simulink model "recordEEGMultiVer"  (R2019a)
settings: Solver=VariableStepAuto  StartTime=0.0  StopTime=1000  RelTol=1e-3
undefined symbols (not defined in the file or in its folder): daq
libraries: dsparch4 x3, commrandsrc3 x3, daqlib x1, dspnetwork x1
settings Model: Creator=Kusunoki  LastModifiedBy=Owner

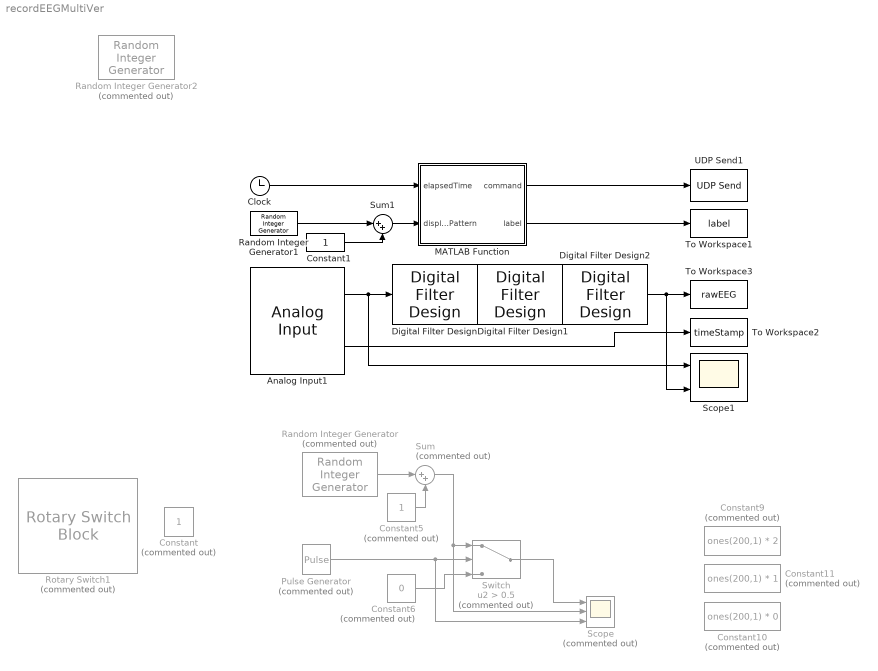
== system recordEEGMultiVer ==
  Analog Input1 : daqlib/Analog Input  DeviceMenu=ni Dev1 (USB-6000)  Device=ni Dev1 (USB-6000)  ObjConstructor=daq.createSession('ni')  NChannelsSelected=8  Channels=1$ai0$$Dev1$1$1$1$1$#1$ai1$$Dev1$1$1$1$1$#1$ai2$$Dev1$1$1$1$1$#1$ai3$$Dev1$1$1$1$1$#1$ai4$$Dev1$1$1$1$1$#1$ai5$$Dev1$1$1$1$1$#1$ai6$$Dev1$1$1$1$1$#1$ai7$$Dev1$1$1$1$1$#  NPorts=1 for all channels  SampleRate=1000  ActualRate=1000  ScansPerTrigger=200  OutputTimestamp=on  AcqMode=0  NumFrameBuffer=100  OutputTriggertime=off
      settings: SourceProductName=Data Acquisition Toolbox  SourceProductBaseCode=DA
  Clock : Clock
  Constant : Constant  Commented=on
  Constant1 : Constant
  Constant10 : Constant  Commented=on  Value=ones(200,1) * 0
  Constant11 : Constant  Commented=on  Value=ones(200,1) * 1
  Constant5 : Constant  Commented=on
  Constant6 : Constant  Commented=on  Value=0
  Constant9 : Constant  Commented=on  Value=ones(200,1) * 2
  Digital Filter Design : dsparch4/Digital Filter Design  mwdsp_browser_bugfix_var=off
  Digital Filter Design1 : dsparch4/Digital Filter Design  mwdsp_browser_bugfix_var=off
  Digital Filter Design2 : dsparch4/Digital Filter Design  mwdsp_browser_bugfix_var=off
  MATLAB Function : MATLAB Function  TreatAsAtomicUnit=on
  Pulse Generator : DiscretePulseGenerator  Commented=on  PulseType=Time based  Period=12  PulseWidth=10/12 * 100
  Random Integer Generator : commrandsrc3/Random Integer Generator  Commented=on  SetSize=2  SeedSource=Auto  Seed=0  SampleTime=12  SamplesPerFrame=1  OutputDataType=uint32  SimulateUsing=Interpreted execution
      settings: SourceProductName=Communications Toolbox
  Random Integer Generator1 : commrandsrc3/Random Integer Generator  SetSize=8  SeedSource=Auto  Seed=0  SampleTime=10  SamplesPerFrame=1  OutputDataType=uint32  SimulateUsing=Interpreted execution
      settings: SourceProductName=Communications Toolbox
  Random Integer Generator2 : commrandsrc3/Random Integer Generator  Commented=on  SetSize=3  SeedSource=Auto  Seed=0  SampleTime=3  SamplesPerFrame=1  OutputDataType=uint32  SimulateUsing=Interpreted execution
      settings: SourceProductName=Communications Toolbox
  Rotary Switch1 : RotarySwitchBlock  Commented=on
      settings: Values={{'0 : Relaxing', '1 : Gripping', '2 : Picking'}, [0 1 2]}
  Scope : Scope  Commented=on  NumInputPorts=3
  Scope1 : Scope  NumInputPorts=2
  Sum : Sum  Commented=on  Inputs=|++
  Sum1 : Sum  Inputs=|++
  Switch : Switch  Commented=on  Criteria=u2 > Threshold  Threshold=0.5
  To Workspace1 : ToWorkspace  VariableName=label  SampleTime=(1/1000) * 200
      settings: Save2DSignal=2-D array (concatenate along first dimension)
  To Workspace2 : ToWorkspace  VariableName=timeStamp  SampleTime=-1
      settings: Save2DSignal=2-D array (concatenate along first dimension)
  To Workspace3 : ToWorkspace  VariableName=rawEEG  SampleTime=-1
      settings: Save2DSignal=2-D array (concatenate along first dimension)
  UDP Send1 : dspnetwork/UDP Send  remoteURL='127.0.0.1'  remotePort=25000  localURL='0.0.0.0'  localPortSource=Automatically determine  localPort=-1  sampletime=-1  blockPlatform=[]  separateLengthPort=0
      settings: SourceProductName=Simulink
  wires:
  MATLAB Function/1(command) -> UDP Send1/1
  Analog Input1/2 -> To Workspace2/1
  MATLAB Function/2(label) -> To Workspace1/1
  Analog Input1/1 -> Scope1/1, Digital Filter Design/1
  Random Integer Generator/1 -> Sum/1
  Constant5/1 -> Sum/2
  Pulse Generator/1 -> Scope/3, Switch/2
  Constant6/1 -> Switch/3
  Switch/1 -> Scope/1
  Sum/1 -> Scope/2, Switch/1
  Digital Filter Design/1 -> Digital Filter Design1/1
  Digital Filter Design1/1 -> Digital Filter Design2/1
  Digital Filter Design2/1 -> Scope1/2, To Workspace3/1
  Clock/1 -> MATLAB Function/1(elapsedTime)
  Random Integer Generator1/1 -> Sum1/1
  Constant1/1 -> Sum1/2
  Sum1/1 -> MATLAB Function/2(displayPattern)

== matlab function recordEEGMultiVer/MATLAB Function ==
  data: elapsedTime input; command output size=1; displayPattern input; label output size=[200,1]
function [command, label] = commandGenerator(elapsedTime,displayPattern)
    command = cast(0,'uint32');
    preDisplayTime = 3;
    displayTime    = 5;
    nonDisplayTime = 2;
    displayPeriod = preDisplayTime + displayTime + nonDisplayTime;
    phase = rem(elapsedTime , displayPeriod);
    if phase < preDisplayTime
        command = cast(displayPattern * 10,'uint32');
        
    elseif phase < (preDisplayTime + displayTime)
        command = cast(displayPattern,'uint32');
        
    elseif phase < (preDisplayTime + displayTime + nonDisplayTime)
        command = cast(0,'uint32');
        
    else 
        %reset to next pattern
        command = cast(0,'uint32');
    end
	
    label = reshape(ones(200,1) * cast(command, 'double'),[200,1]);
end
